simulink model "AttitudeComplementary2"  (Simulink 6.6)
settings: Solver=ode4  StartTime=0.0  StopTime=80  FixedStep=SampleT  RelTol=1e-3
InitFcn:
  | clc
  | Taxi_Var_new
  | failures
  | insInit
  | piccolo_init
values from neighbouring files (symbols this model uses):
  A1 = 0    [Taxi_Var.m]    (also in Taxi_Var_new.m = 0.007)
  Apolar = 0.0899    [Taxi_Var.m]    (also in Taxi_Var_new.m = 0.057)
  APtsamp = 0.005    [failures.m]    (also in piccolo_init.m = 0.05)
  CD0 = 0.0219    [Taxi_Var.m]    (also in Taxi_Var_new.m = 0.022)
  chord = S/span    (= 0.384036716878)    [Taxi_Var.m]    (also in Taxi_Var_new.m = 0.351341681574)
  CL0 = 0.1857    [Taxi_Var.m]    (also in Taxi_Var_new.m = 0.38)
  CLa = 4.6206    [Taxi_Var.m]    (also in Taxi_Var_new.m = 18.5)
  CLa_dot = 1.93    [Taxi_Var.m]    (also in Taxi_Var_new.m = 2.64)
  Clb = -0.0043    [Taxi_Var.m]    (also in Taxi_Var_new.m = -0.06)
  ClDa = 0.1695    [Taxi_Var.m]    (also in Taxi_Var_new.m)
  CLDe = 0.4032    [Taxi_Var.m]    (also in Taxi_Var_new.m = 0.24)
  CLDf = 0.047    [Taxi_Var.m]    (also in Taxi_Var_new.m = 0.4)
  ClDr = 0.0003    [Taxi_Var.m]    (also in Taxi_Var_new.m = 0.055)
  Clp = -0.4425    [Taxi_Var.m]    (also in Taxi_Var_new.m = -0.88)
  CLq = 8.7465    [Taxi_Var.m]    (also in Taxi_Var_new.m = 7.4)
  Clr = 0.0675    [Taxi_Var.m]    (also in Taxi_Var_new.m = 0.04)
  Cm0 = -0.0902    [Taxi_Var.m]    (also in Taxi_Var_new.m = 0.56)
  Cma = -1.3995    [Taxi_Var.m]    (also in Taxi_Var_new.m = -1.58)
  CmDe = -0.9493    [Taxi_Var.m]    (also in Taxi_Var_new.m = -41)
  CmDf = -.021    (= -0.021)    [Taxi_Var.m]    (also in Taxi_Var_new.m)
  Cmq = -10.8760    (= -10.876)    [Taxi_Var.m]    (also in Taxi_Var_new.m = -12)
  Cnb = 0.0281    [Taxi_Var.m]    (also in Taxi_Var_new.m = 0.73)
  CnDa = -0.0031    [Taxi_Var.m]    (also in Taxi_Var_new.m = -0.032)
  CnDr = -0.0882    [Taxi_Var.m]    (also in Taxi_Var_new.m = 0.19)
  Cnp = -0.0695    [Taxi_Var.m]    (also in Taxi_Var_new.m = -0.1)
  Cnr = -0.1045    [Taxi_Var.m]    (also in Taxi_Var_new.m = -0.23)
  CYb = -0.1999    [Taxi_Var.m]    (also in Taxi_Var_new.m = -0.98)
  CYDr = 0.0192    [Taxi_Var.m]    (also in Taxi_Var_new.m = 0.066)
  damax = 25*deg2rad    (= 0.436332312999)    [Taxi_Var.m]    (also in piccolo_init.m)
  damin = -25*deg2rad    (= -0.436332312999)    [Taxi_Var.m]    (also in piccolo_init.m)
  datrim = 0*deg2rad    (= 0)    [Taxi_Var.m]    (also in piccolo_init.m)
  demax = 15*deg2rad    (= 0.261799387799)    [Taxi_Var.m]    (also in piccolo_init.m)
  demin = -15*deg2rad    (= -0.261799387799)    [Taxi_Var.m]    (also in piccolo_init.m)
  detrim = -2.4137*deg2rad    (= -0.0421270121554)    [Taxi_Var.m]    (also in piccolo_init.m = -0.01308996939)
  dfland = 30*deg2rad    (= 0.523598775598)    [Taxi_Var.m]    (also in piccolo_init.m)
  dfmax = 30*deg2rad    (= 0.523598775598)    [Taxi_Var.m]    (also in piccolo_init.m)
  dfmin = 0*deg2rad    (= 0)    [Taxi_Var.m]    (also in piccolo_init.m)
  drmax = 25*deg2rad    (= 0.436332312999)    [Taxi_Var.m]    (also in piccolo_init.m)
  drmin = -25*deg2rad    (= -0.436332312999)    [Taxi_Var.m]    (also in piccolo_init.m)
  drtrim = 0*deg2rad    (= 0)    [Taxi_Var.m]    (also in piccolo_init.m)
  dtmax = 1    [Taxi_Var.m]    (also in piccolo_init.m)
  dtmin = 0    [Taxi_Var.m]    (also in piccolo_init.m)
  dttrim = 0.0725    [Taxi_Var.m]    (also in piccolo_init.m = 0.35)
  Euler_0 = [0; 0; 45]'*pi/180    [Taxi_Var.m]    (also in Taxi_Var_new.m = [0 0 45]'*pi/180)
  heightDown = 0    [insInit.m]
  heightUp = 3000    [insInit.m]
  IdxCmdOrbitRadius = 17    [piccolo_init.m]
  IdxCmdOrbitSense = 18    [piccolo_init.m]
  IdxCmdWp1Alt = 13    [piccolo_init.m]
  IdxCmdWp1Lat = 11    [piccolo_init.m]
  IdxCmdWp1Lon = 12    [piccolo_init.m]
  IdxCmdWp2Alt = 16    [piccolo_init.m]
  IdxCmdWp2Lat = 14    [piccolo_init.m]
  IdxCmdWp2Lon = 15    [piccolo_init.m]
  IdxEstimReserved1 = 4    [piccolo_init.m]
  IdxEstimWEast = 3    [piccolo_init.m]
  IdxEstimWNorth = 2    [piccolo_init.m]
  IdxGainsAltD = 10    [piccolo_init.m]
  IdxGainsAltI = 9    [piccolo_init.m]
  IdxGainsAltP = 8    [piccolo_init.m]
  IdxGainsPdynD = 4    [piccolo_init.m]
  IdxGainsPdynI = 3    [piccolo_init.m]
  IdxGainsPdynP = 2    [piccolo_init.m]
  IdxGainsPitchD = 7    [piccolo_init.m]
  IdxGainsPitchI = 6    [piccolo_init.m]
  IdxGainsPitchP = 5    [piccolo_init.m]
  IdxGainsRollD = 17    [piccolo_init.m]
  IdxGainsRollI = 16    [piccolo_init.m]
  IdxGainsRollP = 15    [piccolo_init.m]
  IdxGainsSlopeElevatorD = 25    [piccolo_init.m]
  IdxGainsSlopeElevatorP = 26    [piccolo_init.m]
  IdxGainsTrackConv = 24    [piccolo_init.m]
  IdxGainsTrackD = 23    [piccolo_init.m]
  IdxGainsTrackI = 22    [piccolo_init.m]
  IdxGainsTrackP = 21    [piccolo_init.m]
  IdxGainsTurnD = 14    [piccolo_init.m]
  IdxGainsTurnI = 13    [piccolo_init.m]
  IdxGainsTurnP = 12    [piccolo_init.m]
  IdxGainsYawD = 20    [piccolo_init.m]
  IdxGainsYawI = 19    [piccolo_init.m]
  IdxGainsYawP = 18    [piccolo_init.m]
  IdxLimitsAileronMax = 11    [piccolo_init.m]
  IdxLimitsAileronMin = 10    [piccolo_init.m]
  IdxLimitsBankMax = 9    [piccolo_init.m]
  IdxLimitsBankMin = 8    [piccolo_init.m]
  IdxLimitsElevatorMax = 13    [piccolo_init.m]
  IdxLimitsElevatorMin = 12    [piccolo_init.m]
  IdxLimitsFlapMax = 19    [piccolo_init.m]
  IdxLimitsFlapMin = 18    [piccolo_init.m]
  IdxLimitsPdynMax = 3    [piccolo_init.m]
  IdxLimitsPdynMin = 2    [piccolo_init.m]
  IdxLimitsRudderMax = 15    [piccolo_init.m]
  IdxLimitsRudderMin = 14    [piccolo_init.m]
  IdxLimitsThrottleMax = 17    [piccolo_init.m]
  IdxLimitsThrottleMin = 16    [piccolo_init.m]
  IdxSensorsAlt = 5    [piccolo_init.m]
  IdxSensorsLat = 3    [piccolo_init.m]
  IdxSensorsLon = 4    [piccolo_init.m]
  IdxSensorsVDown = 8    [piccolo_init.m]
  IdxSensorsVEast = 7    [piccolo_init.m]
  IdxSensorsVNorth = 6    [piccolo_init.m]
  IdxStatesGlobal = 2    [piccolo_init.m]
  IdxStatesManual = 16    [piccolo_init.m]
  IdxStatesMode = 15    [piccolo_init.m]
  ISA_g = 9.815    [Taxi_Var.m]    (also in Taxi_Var_new.m)
  ISA_hmax = 2000    [Taxi_Var.m]    (also in Taxi_Var_new.m)
  ISA_lapse = .0065    (= 0.0065)    [Taxi_Var.m]    (also in Taxi_Var_new.m)
  ISA_P0 = 101325    [Taxi_Var.m]    (also in Taxi_Var_new.m)
  ISA_R = 287    [Taxi_Var.m]    (also in Taxi_Var_new.m)
  ISA_rho0 = 1.225    [Taxi_Var.m]    (also in Taxi_Var_new.m)
  ISA_T0 = 289    [Taxi_Var.m]    (also in Taxi_Var_new.m)
  Ixx = 3.689084    [Taxi_Var.m]    (also in Taxi_Var_new.m = 3.8)
  Iyy = 7.43789    [Taxi_Var.m]    (also in Taxi_Var_new.m = 9.58)
  Izz = 10.22202    [Taxi_Var.m]    (also in Taxi_Var_new.m = 9.68)
  latDown = -100000    [insInit.m]
  latUp = 100000    [insInit.m]
  lonDown = -100000    [insInit.m]
  lonUp = 100000    [insInit.m]
  mass = 22.5    [Taxi_Var.m]    (also in Taxi_Var_new.m = 8.16466266)
  MinThK = 0.075    [Taxi_Var.m]    (also in Taxi_Var_new.m = 0.077)
  ... (+8 more)
undefined symbols (not defined in the file or in its folder): clock, DiscIntNeverNeededParam, Earth, gaind, polesd, WGS84, zerosd
libraries: piccolo_library x60, simulink x51, aerolibconvert2 x14, dspsigops x5, aerolibasang x5, aerolibatmos2 x2, aerolibtransform2 x2, aerolibnav x2, dspmtrx3 x1, aerolibutil x1
(part 1 of 6)
CloseFcn:
  | rtwprivate ssgencode ModelCloseRequest AttitudeComplementary
settings Model: Creator=ASL_Lab  LastModifiedBy=ASL_Lab
settings DebuggingCC: MultiTaskDSMMsg=warning  MultiTaskCondExecSysMsg=none  StrictBusMsg=None
settings HardwareCC: TargetHWDeviceType=32-bit Generic
settings RTWCC: IncludeERTFirstTime=on

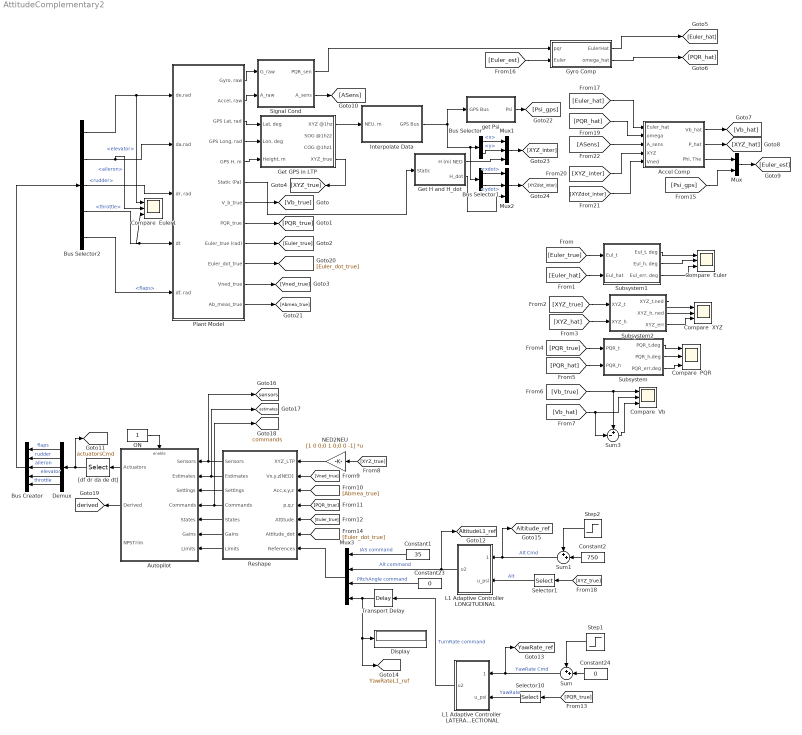
== system AttitudeComplementary2 ==
  Accel Comp : Subsystem
  Autopilot : Subsystem  Orientation=left
  Bus Creator : BusCreator  Orientation=left  Inputs=5
  Bus Selector : BusSelector  OutputSignals=x,y
  Bus Selector1 : BusSelector  OutputSignals=xdot,ydot
  Bus Selector2 : BusSelector  OutputSignals=elevator,aileron,rudder,throttle,flaps
  Compare  Euler : Scope  NumInputPorts=3
      settings: TimeRange=80  YMin=-20~-58.03108808290165~-7.51142166084415  YMax=31.19170984455958~41.45077720207246~7.726417629669186  SaveName=ScopeData20
  Compare  Euler1 : Scope  NumInputPorts=3
      settings: TimeRange=100  YMin=-0.275~-1~0.675  YMax=0.275~1~1  SaveName=ScopeData19
  Compare  PQR : Scope  NumInputPorts=3
      settings: TimeRange=200  YMin=-50~-350000~-450000  YMax=55~450000~350000  SaveName=ScopeData8
  Compare  Vb : Scope  NumInputPorts=3
      settings: TimeRange=1200  YMin=-5~-4.608235729481237~-0.2140564617663046  YMax=35~22.0134426214664~0.2078550324478208  SaveName=ScopeData12
  Compare  XYZ : Scope  NumInputPorts=3
      settings: TimeRange=70  YMin=-1000~-1000~-2.5  YMax=1200~1200~4  SaveName=ScopeData2
  Constant1 : Constant  Orientation=left  Value=35
  Constant2 : Constant  Orientation=left  Value=750
  Constant23 : Constant  Orientation=left  Value=0
  Constant24 : Constant  Orientation=left  Value=0
  Demux : Demux  Orientation=left  Outputs=5
  Display : Display
  Get GPS in LTP : Subsystem
  "Get H and H_dot " : Subsystem
  Gyro Comp : Subsystem
  Interpolate Data : Subsystem
  L1 Adaptive Controller LATERAL-DIRECTIONAL : Subsystem  Orientation=left  mask{gamma=-2000, m=4, omega=2, Pbound=.1, L1ONOFF=0}
      mask prompts: gamma "L1 gain"; m "state predictor (m)"; omega "low-pass filter (omega)"; Pbound "projection bounds"; L1ONOFF "L1 switch"
  L1 Adaptive Controller LONGITUDINAL : Subsystem  Orientation=left  mask{gamma=-1, m=4, omega=1, Pbound=50, L1ONOFF=0}
      mask prompts: gamma "L1 gain"; m "state predictor (m)"; omega "low-pass filter (omega)"; Pbound "projection bounds"; L1ONOFF "L1 switch"
  Mux : Mux  Inputs=2
  Mux1 : Mux  Inputs=3
  Mux2 : Mux  Inputs=3
  Mux3 : Mux  Orientation=left
  NED2NEU : Gain  Orientation=left  Gain=[1 0 0;0 1 0;0 0 -1]  Multiplication=Matrix(K*u)  SaturateOnIntegerOverflow=on
  ON : Constant
  Plant Model : Subsystem
  Reshape : Subsystem  Orientation=left
  Selector1 : Selector  Orientation=left  IndexOptions=Index vector (dialog)  Indices=3  OutputSizes=1  InputPortWidth=3
  Selector10 : Selector  Orientation=left  IndexOptions=Index vector (dialog)  Indices=3  OutputSizes=1  InputPortWidth=3
  Signal Cond : Subsystem
  Step1 : Step  Orientation=left  Time=2  After=0  SampleTime=0
  Step2 : Step  Orientation=left  Time=35  After=-250  SampleTime=0
  Subsystem : Subsystem
  Subsystem1 : Subsystem
  Subsystem2 : Subsystem
  Sum : Sum  Orientation=left  Inputs=++|  SaturateOnIntegerOverflow=on
  Sum1 : Sum  Orientation=left  Inputs=++|  SaturateOnIntegerOverflow=on
  Sum3 : Sum  Inputs=+-|
  Transport Delay : TransportDelay  Orientation=left  DelayTime=tdelay
  "[df dr da de dt]" : Selector  Orientation=left  IndexOptions=Index vector (dialog)  Indices=[10 6 2 4 8]  OutputSizes=[(-2)]  InputPortWidth=12
  get Psi : Subsystem
  tag scope: AltitudeL1_ref=global, Altitude_ref=global, YawRateL1_ref=global, YawRate_ref=global, actuatorsCmd=global, commands=global, derived=global, estimates=global, sensors=global
  wires:
  Plant Model/1("Gyro, raw") -> Signal Cond/1(G_raw)
  Plant Model/2("Accel, raw") -> Signal Cond/2(A_raw)
  Plant Model/3("GPS Lat, rad") -> Get GPS in LTP/1("Lat, deg")
  Plant Model/5("GPS H, m") -> Get GPS in LTP/3("Height, m")
  Plant Model/4("GPS Long, rad") -> Get GPS in LTP/2("Lon, deg")
  Signal Cond/1(PQR_sen) -> Gyro Comp/1(pqr)
  Gyro Comp/1(EulerHat) -> [Euler_hat]
  Accel Comp/3("Phi, The") -> Mux/1
  Get GPS in LTP/1(XYZ @1hz) -> Interpolate Data/1(NEU. m)
  Gyro Comp/2(omega_hat) -> [PQR_hat]
  Bus Selector/1 -> Mux1/1  "<x>"
  Bus Selector/2 -> Mux1/2  "<y>"
  Bus Selector1/1 -> Mux2/1  "<xdot>"
  Bus Selector1/2 -> Mux2/2  "<ydot>"
  Plant Model/7(V_b_true) -> [Vb_true]
  Plant Model/8(PQR_true) -> [PQR_true]
  Plant Model/9(Euler_true (rad)) -> [Euler_true]
  Plant Model/11(Vned_true) -> [Vned_true]
  Accel Comp/1(Vb_hat) -> [Vb_hat]
  Accel Comp/2(P_hat) -> [XYZ_hat]
  Subsystem1/1("Eul_t, deg") -> Compare  Euler/1
  Subsystem1/2("Eul_h, deg") -> Compare  Euler/2
  Subsystem1/3("Eul_err, deg") -> Compare  Euler/3
  [XYZ_true] -> Subsystem2/1(XYZ_t)
  [XYZ_hat] -> Subsystem2/2(XYZ_h)
  Subsystem/1(PQR_t,deg) -> Compare  PQR/1
  Subsystem/2(PQR_h,deg) -> Compare  PQR/2
  Subsystem/3(PQR_err,deg) -> Compare  PQR/3
  [Vb_true] -> Compare  Vb/1, Sum3/1
  [Vb_hat] -> Sum3/2, Compare  Vb/2
  Sum3/1 -> Compare  Vb/3
  Get GPS in LTP/4(XYZ_true) -> [XYZ_true]
  [PQR_true] -> Subsystem/1(PQR_t)
  [PQR_hat] -> Subsystem/2(PQR_h)
  [Euler_true] -> Subsystem1/1(Eul_t)
  [Euler_hat] -> Subsystem1/2(Eul_hat)
  Subsystem2/1(XYZ_t,ned) -> Compare  XYZ/1
  Subsystem2/2("XYZ_h, ned") -> Compare  XYZ/2
  Subsystem2/3(XYZ_err) -> Compare  XYZ/3
  "Get H and H_dot "/1(H (m) NED) -> Mux1/3
  "Get H and H_dot "/2(H_dot) -> Mux2/3
  [XYZ_true] -> NED2NEU/1
  [Vned_true] -> Reshape/2(Vx,y,z[NED])
  [Abmea_true] -> Reshape/3(Acc,x,y,z)
  [PQR_true] -> Reshape/4(p,q,r)
  Reshape/1(Sensors) -> Autopilot/1(Sensors), [sensors]
  Reshape/2(Estimates) -> Autopilot/2(Estimates), [estimates]
  Reshape/3(Settings) -> Autopilot/3(Settings)
  Reshape/4(Commands) -> Autopilot/4(Commands), [commands]
  Reshape/5(States) -> Autopilot/5(States)
  Reshape/6(Gains) -> Autopilot/6(Gains)
  Reshape/7(Limits) -> Autopilot/7(Limits)
  ON/1 -> Autopilot/Enable
  Autopilot/1(Actuators) -> "[df dr da de dt]"/1
  "[df dr da de dt]"/1 -> Demux/1, [actuatorsCmd]
  [Euler_true] -> Reshape/5(Attitude)
  [Euler_dot_true] -> Reshape/6(Attitude_dot)
  Autopilot/2(Derived) -> [derived]
  Constant1/1 -> Mux3/1  "IAS command"
  L1 Adaptive Controller LONGITUDINAL/1(u2) -> [AltitudeL1_ref], Mux3/2  "Alt command"
  Constant23/1 -> Mux3/3  "PitchAngle command"
  L1 Adaptive Controller LATERAL-DIRECTIONAL/1(u2) -> Transport Delay/1  "TurnRate command"
  Mux3/1 -> Reshape/7(References)
  Sum/1 -> L1 Adaptive Controller LATERAL-DIRECTIONAL/1(u_psi_c), [YawRate_ref]  "YawRate Cmd"
  [PQR_true] -> Selector10/1
  Selector10/1 -> L1 Adaptive Controller LATERAL-DIRECTIONAL/2(u_psi)  "YawRate"
  Constant24/1 -> Sum/2
  Step1/1 -> Sum/1
  Transport Delay/1 -> Mux3/4, Display/1, [YawRateL1_ref]
  Sum1/1 -> [Altitude_ref], L1 Adaptive Controller LONGITUDINAL/1(u_psi_c)  "Alt Cmd"
  Constant2/1 -> Sum1/2
  Step2/1 -> Sum1/1
  [XYZ_true] -> Selector1/1
  Selector1/1 -> L1 Adaptive Controller LONGITUDINAL/2(u_psi)  "Alt"
  Demux/1 -> Bus Creator/1  "flaps"
  Demux/2 -> Bus Creator/2  "rudder"
  Demux/3 -> Bus Creator/3  "aileron"
  Demux/4 -> Bus Creator/4  "elevator"
  Demux/5 -> Bus Creator/5  "throttle"
  Bus Creator/1 -> Bus Selector2/1
  Bus Selector2/1 -> Plant Model/1(de,rad), Compare  Euler1/1  "<elevator>"
  Bus Selector2/2 -> Plant Model/2(da,rad), Compare  Euler1/2  "<aileron>"
  Bus Selector2/3 -> Plant Model/3("dr, rad")  "<rudder>"
  Bus Selector2/4 -> Compare  Euler1/3, Plant Model/4(dt)  "<throttle>"
  Bus Selector2/5 -> Plant Model/5("df, rad")  "<flaps>"
  Plant Model/10(Euler_dot_true) -> [Euler_dot_true]
  Plant Model/12(Ab_meas_true) -> [Abmea_true]
  Mux/1 -> [Euler_est]
  Plant Model/6(Static (Pa)) -> "Get H and H_dot "/1(Static)
  Interpolate Data/1(GPS Bus) -> Bus Selector/1, Bus Selector1/1, get Psi/1(GPS Bus)
  get Psi/1(Psi) -> [Psi_gps]
  Mux1/1 -> [XYZ_inter]
  Mux2/1 -> [XYZdot_inter]
  [Psi_gps] -> Mux/2
  [Euler_est] -> Gyro Comp/2(Euler)
  [Euler_hat] -> Accel Comp/1(Euler_hat)
  [PQR_hat] -> Accel Comp/2(omega)
  [XYZ_inter] -> Accel Comp/4(XYZ)
  [XYZdot_inter] -> Accel Comp/5(Vned)
  Signal Cond/2(A_sens) -> [ASens]
  [ASens] -> Accel Comp/3(A_sens)
  NED2NEU/1 -> Reshape/1(XYZ_LTP)

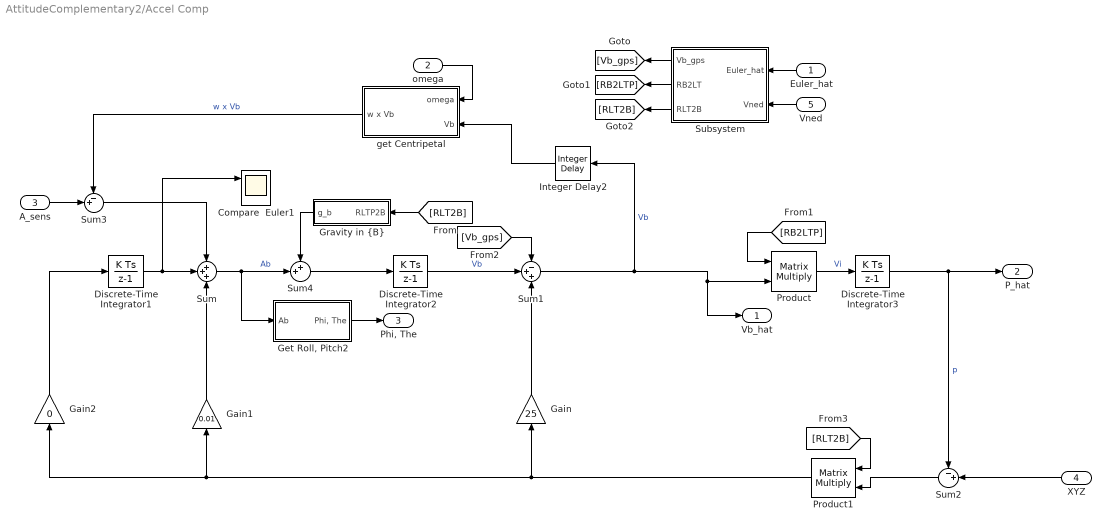
== system AttitudeComplementary2/Accel Comp ==
  Euler_hat : Inport  Orientation=left
  omega : Inport  Port=2
  A_sens : Inport  Port=3
  XYZ : Inport  Orientation=left  Port=4
  Vned : Inport  Orientation=left  Port=5
  Compare  Euler1 : Scope  NumInputPorts=3
      settings: TimeRange=80  YMin=-20~-200~-7.51142166084415  YMax=60~200~7.726417629669186  SaveName=ScopeData23
  Discrete-Time Integrator1 : DiscreteIntegrator  SampleTime=SampleT  ICPrevOutput=DiscIntNeverNeededParam  ICPrevScaledInput=DiscIntNeverNeededParam
  Discrete-Time Integrator2 : DiscreteIntegrator  InitialCondition=Vb_0  SampleTime=SampleT  ICPrevOutput=DiscIntNeverNeededParam  ICPrevScaledInput=DiscIntNeverNeededParam
  Discrete-Time Integrator3 : DiscreteIntegrator  InitialCondition=[Pos_0(1) Pos_0(2) -Pos_0(3)]  SampleTime=SampleT  ICPrevOutput=DiscIntNeverNeededParam  ICPrevScaledInput=DiscIntNeverNeededParam
  Gain : Gain  Orientation=up  Gain=25
  Gain1 : Gain  Orientation=up  Gain=0.01
  Gain2 : Gain  Orientation=up  Gain=0
  "Get Roll, Pitch2" : Subsystem
  "Gravity in {B}" : Subsystem  Orientation=left
  Integer Delay2 : simulink/Discrete/Integer Delay  Orientation=left  vinit=0.0  samptime=-1  NumDelays=1
  Product : Product  Multiplication=Matrix(*)  RndMeth=Zero
  Product1 : Product  Orientation=left  Multiplication=Matrix(*)  RndMeth=Zero
  Subsystem : Subsystem  Orientation=left
  Sum : Sum  Inputs=+++
  Sum1 : Sum  Inputs=-++
  Sum2 : Sum  Orientation=left  Inputs=-+|
  Sum3 : Sum  Inputs=-+|
  Sum4 : Sum  Inputs=++|
  get Centripetal : Subsystem  Orientation=left
  Vb_hat : Outport
  P_hat : Outport  Port=2
  "Phi, The" : Outport  Port=3
  wires:
  Sum2/1 -> Product1/2
  Discrete-Time Integrator3/1 -> Sum2/1, P_hat/1  "p"
  Discrete-Time Integrator1/1 -> Sum/2, Compare  Euler1/1
  Discrete-Time Integrator2/1 -> Sum1/2  "Vb"
  "Get Roll, Pitch2"/1("Phi, The") -> "Phi, The"/1
  A_sens/1 -> Sum3/2
  omega/1 -> get Centripetal/1(omega)
  Euler_hat/1 -> Subsystem/1(Euler_hat)
  Vned/1 -> Subsystem/2(Vned)
  Product/1 -> Discrete-Time Integrator3/1  "Vi"
  Sum1/1 -> Integer Delay2/1, Product/2, Vb_hat/1  "Vb"
  XYZ/1 -> Sum2/2
  Subsystem/1(Vb_gps) -> [Vb_gps]
  Subsystem/2(RB2LT) -> [RB2LTP]
  Subsystem/3(RLT2B) -> [RLT2B]
  [RLT2B] -> "Gravity in {B}"/1(RLTP2B)
  [RB2LTP] -> Product/1
  [Vb_gps] -> Sum1/1
  [RLT2B] -> Product1/1
  Product1/1 -> Gain2/1, Gain1/1, Gain/1
  Gain2/1 -> Discrete-Time Integrator1/1
  Gain1/1 -> Sum/3
  Gain/1 -> Sum1/3
  Sum3/1 -> Sum/1
  Sum4/1 -> Discrete-Time Integrator2/1
  "Gravity in {B}"/1(g_b) -> Sum4/1
  Sum/1 -> Sum4/2, "Get Roll, Pitch2"/1(Ab)  "Ab"
  Integer Delay2/1 -> get Centripetal/2(Vb)
  get Centripetal/1(w x Vb) -> Sum3/1  "w x Vb"

== system AttitudeComplementary2/Autopilot ==
  Sensors : Inport  PortDimensions=SizeSensors
  Estimates : Inport  Port=2  PortDimensions=SizeEstim
  Settings : Inport  Port=3  PortDimensions=SizeSet
  Commands : Inport  Port=4  PortDimensions=SizeCmd
  States : Inport  Port=5  PortDimensions=SizeStates
  Gains : Inport  Port=6  PortDimensions=SizeGains
  Limits : Inport  Port=7  PortDimensions=SizeLimits
  Autopilot Enable : EnablePort  StatesWhenEnabling=reset
  Air System Vector Inputs : piccolo_library/Flight Mechanics/Air System Vector Inputs  SystemSampleTime=-1  tsamp=APtsamp
  Altitude Control Vector Inputs : Subsystem  AncestorBlock=piccolo_library/Controllers/Longitudinal/Altitude Control Vector Inputs  mask(Altitude controller){tsamp=APtsamp}
      mask prompts: tsamp "Sample time:"
      mask help: The system computes the throttle command required for maintaining a specified altitude.
  Demux{,1..6} (7 alike) : Demux  Outputs=7
  Flap Control Vector Inputs : Subsystem  mask(Flap controller){tsamp=APtsamp}
      mask prompts: tsamp "Sample time:"
      mask help: The system provides the flap command.
  Gain : Gain  SaturateOnIntegerOverflow=on
  Gain1 : Gain  SaturateOnIntegerOverflow=on
  Guidance & Navigation Vector Input : Subsystem  AncestorBlock=piccolo_library/Controllers/Guidance/Guidance & Navigation Vector Input  mask(Guidance and Navigation){tsamp=1, aptsamp=APtsamp}
      mask prompts: tsamp "Guidance sample time:"; aptsamp "Autopilot sample time:"
      mask help: Steer the airplane to track a flightplan or to loiter around a single waypoint.
  Mux : Mux  Inputs=12
  Mux1 : Mux  Inputs=5
  Mux2 : Mux  Inputs=7
  Pitch Control  Vector Inputs : Subsystem  AncestorBlock="piccolo_library/Controllers/Longitudinal/Pitch Control  Vector Inputs"  mask(Pitch Control){tsamp=APtsamp}
      mask prompts: tsamp "Sample time:"
      mask help: The pitch controller includes pitch angle hold, dynamic pressure hold, and turn compensation.
  Reserved Outputs : Constant  Value=0
  Roll Control Vector Inputs : Subsystem  AncestorBlock=piccolo_library/Controllers/Lateral/Roll Control Vector Inputs  mask(Roll Control){tsamp=APtsamp}
      mask prompts: tsamp "Sample time:"
      mask help: Roll controller using bank angle hold and turn rate hold.
  Yaw Control Vector Inputs : Subsystem  AncestorBlock=piccolo_library/Controllers/Lateral/Yaw Control Vector Inputs  mask(Yaw Control){tsamp=APtsamp}
      mask prompts: tsamp "Sample time:"
      mask help: Yaw controller using PID loops and actuator output saturation.
  Actuators : Outport  OutDataType=fixdt(1,16,0)  OutScaling=[]
  Derived : Outport  Port=2  OutDataType=fixdt(1,16,0)  OutScaling=[]
  NPSTrim : Outport  Port=3  OutDataType=fixdt(1,16,0)  OutScaling=[]
  wires:
  Mux/1 -> Gain/1, NPSTrim/1
  Mux1/1 -> Roll Control Vector Inputs/8(Derived), Altitude Control Vector Inputs/8(Derived), Pitch Control  Vector Inputs/8(Derived), Guidance & Navigation Vector Input/8(Derived), Yaw Control Vector Inputs/8(Derived), Air System Vector Inputs/8, Flap Control Vector Inputs/8(Derived), Gain1/1
  Roll Control Vector Inputs/1(Actuator) -> Mux/2
  Pitch Control  Vector Inputs/1(Actuator) -> Mux/4
  Altitude Control Vector Inputs/1(Actuator) -> Mux/8
  Sensors/1 -> Mux2/1
  Estimates/1 -> Mux2/2
  Settings/1 -> Mux2/3
  Commands/1 -> Mux2/4
  States/1 -> Mux2/5
  Gains/1 -> Mux2/6
  Limits/1 -> Mux2/7
  Demux/1 -> Altitude Control Vector Inputs/1(Sensors)
  Demux/2 -> Altitude Control Vector Inputs/2(Estimates)
  Demux/3 -> Altitude Control Vector Inputs/3(Settings)
  Demux/4 -> Altitude Control Vector Inputs/4(Commands)
  Demux/5 -> Altitude Control Vector Inputs/5(States)
  Demux/6 -> Altitude Control Vector Inputs/6(Gains)
  Demux/7 -> Altitude Control Vector Inputs/7(Limits)
  Demux1/1 -> Roll Control Vector Inputs/1(Sensors)
  Demux1/2 -> Roll Control Vector Inputs/2(Estimates)
  Demux1/3 -> Roll Control Vector Inputs/3(Settings)
  Demux1/4 -> Roll Control Vector Inputs/4(Commands)
  Demux1/5 -> Roll Control Vector Inputs/5(States)
  Demux1/6 -> Roll Control Vector Inputs/6(Gains)
  Demux1/7 -> Roll Control Vector Inputs/7(Limits)
  Demux2/1 -> Pitch Control  Vector Inputs/1(Sensors)
  Demux2/2 -> Pitch Control  Vector Inputs/2(Estimates)
  Demux2/3 -> Pitch Control  Vector Inputs/3(Settings)
  Demux2/4 -> Pitch Control  Vector Inputs/4(Commands)
  Demux2/5 -> Pitch Control  Vector Inputs/5(States)
  Demux2/6 -> Pitch Control  Vector Inputs/6(Gains)
  Demux2/7 -> Pitch Control  Vector Inputs/7(Limits)
  Demux3/1 -> Guidance & Navigation Vector Input/1(Sensors)
  Demux3/2 -> Guidance & Navigation Vector Input/2(Estimates)
  Demux3/3 -> Guidance & Navigation Vector Input/3(Settings)
  Demux3/4 -> Guidance & Navigation Vector Input/4(Commands)
  Demux3/5 -> Guidance & Navigation Vector Input/5(States)
  Demux3/6 -> Guidance & Navigation Vector Input/6(Gains)
  Demux3/7 -> Guidance & Navigation Vector Input/7(Limits)
  Demux4/1 -> Yaw Control Vector Inputs/1(Sensors)
  Demux4/2 -> Yaw Control Vector Inputs/2(Estimates)
  Demux4/3 -> Yaw Control Vector Inputs/3(Settings)
  Demux4/4 -> Yaw Control Vector Inputs/4(Commands)
  Demux4/5 -> Yaw Control Vector Inputs/5(States)
  Demux4/6 -> Yaw Control Vector Inputs/6(Gains)
  Demux4/7 -> Yaw Control Vector Inputs/7(Limits)
  Demux5/1 -> Air System Vector Inputs/1
  Demux5/2 -> Air System Vector Inputs/2
  Demux5/3 -> Air System Vector Inputs/3
  Demux5/4 -> Air System Vector Inputs/4
  Demux5/5 -> Air System Vector Inputs/5
  Demux5/6 -> Air System Vector Inputs/6
  Demux5/7 -> Air System Vector Inputs/7
  Mux2/1 -> Demux1/1, Demux/1, Demux2/1, Demux3/1, Demux4/1, Demux5/1, Demux6/1
  Reserved Outputs/1 -> Mux/11, Mux/9, Mux/7, Mux/1, Mux/3, Mux/5, Mux/12
  Yaw Control Vector Inputs/1(Actuator) -> Mux/6
  Flap Control Vector Inputs/1(Actuator) -> Mux/10
  Demux6/1 -> Flap Control Vector Inputs/1(Sensors)
  Demux6/2 -> Flap Control Vector Inputs/2(Estimates)
  Demux6/3 -> Flap Control Vector Inputs/3(Settings)
  Demux6/4 -> Flap Control Vector Inputs/4(Commands)
  Demux6/5 -> Flap Control Vector Inputs/5(States)
  Demux6/6 -> Flap Control Vector Inputs/6(Gains)
  Demux6/7 -> Flap Control Vector Inputs/7(Limits)
  Air System Vector Inputs/1 -> Mux1/1
  Roll Control Vector Inputs/2(Param) -> Mux1/2
  Pitch Control  Vector Inputs/2(Param) -> Mux1/3
  Guidance & Navigation Vector Input/1(Param) -> Mux1/4
  Altitude Control Vector Inputs/2(Param) -> Mux1/5
  Gain/1 -> Actuators/1
  Gain1/1 -> Derived/1

== system AttitudeComplementary2/Get GPS in LTP ==
  "Lat, deg" : Inport
  "Lon, deg" : Inport  Port=2
  "Height, m" : Inport  Port=3
  Angle Conversion : aerolibconvert2/Angle Conversion  SystemSampleTime=-1  IU=rad  OU=deg
  Angle Conversion1 : aerolibconvert2/Angle Conversion  SystemSampleTime=-1  IU=rad  OU=deg
  Angle Conversion2 : aerolibconvert2/Angle Conversion  SystemSampleTime=-1  IU=rad  OU=deg
  Constant : Constant  Orientation=left  Value=[0 , 37.0004768371582, -122.061897277832]
  Demux : Demux  Outputs=3
  Demux1 : Demux  Outputs=3
  Discrete Derivative : simulink/Discrete/Discrete Derivative  SystemSampleTime=-1  gainval=1.0  ICPrevScaledInput=0.0  OutDataType=sfix(16)  OutScaling=2^-10  DoSatur=off
  Fcn : Fcn  Expr=sqrt(u(1)^2+u(2)^2+u(3)^2)
  Geod2LTP2 : Subsystem
      mask Description:
      | This block provides transformation of the Geodetic coordinates
      | to the LTP coorinate system. The block uses two consecutive transformations
      | (Geodetic -> ECEF ->LTP).
      | Geodetic coordinates of the LTP origin should also be predetermined.
      mask Help: Oops!
      mask Display: plot(0,0,100,100,[45,40,35,40,40],[85,95,85,95,40],[85,95,85,95,40],[35,40,45,40,40],[60,40,10,20,10,14],[70,40,10,13,10,20],[56,45],[70,70],[60,60],[50,60],[60,60],[30,40],[50,60],[20,20],[30,40],[20,20],[45,55],[35,25],[75,65],[35,25])
  Mux : Mux  Inputs=3
  NED2NEU : Gain  Gain=[1 0 0;0 1 0;0 0 -1]  Multiplication=Matrix(K*u)  SaturateOnIntegerOverflow=on
  Reshape1 : Reshape
  Sim Latency : Subsystem
  Sim Latency3 : Subsystem
  Sim Latency4 : Subsystem
  Sim Latency5 : Subsystem
  Sim Latency6 : Subsystem
  Trigonometric Function : Trigonometry  Operator=atan2
  XYZ @1hz : Outport
  SOG @1hz2 : Outport  Port=2
  COG @1hz1 : Outport  Port=3
  XYZ_true : Outport  Port=4
  wires:
  Constant/1 -> Geod2LTP2/1("Height, Lat, Lon Initials from GPS")
  Geod2LTP2/1("NEU, m") -> Demux1/1, Discrete Derivative/1, Reshape1/1
  "Lat, deg"/1 -> Angle Conversion1/1
  "Lon, deg"/1 -> Angle Conversion2/1
  "Height, m"/1 -> Geod2LTP2/4(Hight,m(GPS))
  Fcn/1 -> Sim Latency6/1(Fast Data)
  Demux/2 -> Trigonometric Function/1
  Demux/1 -> Trigonometric Function/2
  Trigonometric Function/1 -> Angle Conversion/1
  Angle Conversion/1 -> Sim Latency5/1(Fast Data)
  Discrete Derivative/1 -> Demux/1, Fcn/1
  Mux/1 -> XYZ @1hz/1
  Angle Conversion1/1 -> Geod2LTP2/2("Lat, deg(GPS)")
  Angle Conversion2/1 -> Geod2LTP2/3("Lon, deg(GPS)")
  Demux1/1 -> Sim Latency/1(Fast Data)
  Demux1/2 -> Sim Latency3/1(Fast Data)
  Demux1/3 -> Sim Latency4/1(Fast Data)
  Sim Latency/1(1Hz Data) -> Mux/1
  Sim Latency3/1(1Hz Data) -> Mux/2
  Sim Latency4/1(1Hz Data) -> Mux/3
  Sim Latency5/1(1Hz Data) -> COG @1hz1/1
  Sim Latency6/1(1Hz Data) -> SOG @1hz2/1
  Reshape1/1 -> NED2NEU/1
  NED2NEU/1 -> XYZ_true/1

== system AttitudeComplementary2/Get H and H_dot  ==
  Static : Inport
  Discrete Derivative : simulink/Discrete/Discrete Derivative  SystemSampleTime=-1  gainval=1.0  ICPrevScaledInput=-0.6  OutDataType=sfix(16)  OutScaling=2^-10  DoSatur=off
  Gain : Gain  Gain=-1
  Pressure Altitude : aerolibatmos2/Pressure Altitude  SystemSampleTime=-1  units=Metric (MKS)  action=Warning
  H (m) NED : Outport
  H_dot : Outport  Port=2
  wires:
  Pressure Altitude/1 -> Gain/1
  Gain/1 -> Discrete Derivative/1, H (m) NED/1
  Discrete Derivative/1 -> H_dot/1
  Static/1 -> Pressure Altitude/1

== system AttitudeComplementary2/Gyro Comp ==
  pqr : Inport
  Euler : Inport  Orientation=left  Port=2
  3vector LPF : Subsystem  mask{flpf=5}
      mask prompts: flpf "LowPass Freq"
      mask Display: droots([],-flpf,flpf)
  Constant : Constant  Value=[1 0 0]
  Discrete-Time Integrator1 : DiscreteIntegrator  SampleTime=SampleT  ICPrevOutput=DiscIntNeverNeededParam  ICPrevScaledInput=DiscIntNeverNeededParam
  Discrete-Time Integrator2 : DiscreteIntegrator  InitialCondition=PQR_0  SampleTime=SampleT  ICPrevOutput=DiscIntNeverNeededParam  ICPrevScaledInput=DiscIntNeverNeededParam
  Discrete-Time Integrator3 : DiscreteIntegrator  InitialCondition=Euler_0  SampleTime=SampleT  ICPrevOutput=DiscIntNeverNeededParam  ICPrevScaledInput=DiscIntNeverNeededParam
  Embedded MATLAB Function : Stateflow chart
  Gain : Gain  Orientation=up  Gain=3
  Gain1 : Gain  Orientation=up  Gain=0.5
  Gain2 : Gain  Orientation=up  Gain=0.01
  Integer Delay : simulink/Discrete/Integer Delay  Orientation=left  vinit=0.0  samptime=-1  NumDelays=1
  Scope1 : Scope
      settings: YMin=-0.08  YMax=0.035  SaveName=ScopeData28
  Slider Gain : simulink/Math Operations/Slider Gain  SystemSampleTime=-1  low=0  gain=0  high=0.09
  Sum : Sum  Inputs=+++
  Sum1 : Sum  Inputs=|++
  Sum2 : Sum  Orientation=left  Inputs=-+|
  Sum3 : Sum  Inputs=|++
  EulerHat : Outport
  omega_hat : Outport  Port=2
  wires:
  Discrete-Time Integrator2/1 -> Sum/2
  Sum1/1 -> Discrete-Time Integrator2/1
  Discrete-Time Integrator1/1 -> Sum1/1, Scope1/1
  Gain/1 -> Sum/3
  Gain1/1 -> Sum1/2
  Gain2/1 -> Discrete-Time Integrator1/1
  Discrete-Time Integrator3/1 -> EulerHat/1, Sum2/1, Integer Delay/1
  Euler/1 -> Sum2/2
  Sum2/1 -> Gain2/1, Gain1/1, Gain/1
  Sum/1 -> Embedded MATLAB Function/2(pqr), 3vector LPF/1(In1)
  Embedded MATLAB Function/1(lamDot) -> Discrete-Time Integrator3/1
  Integer Delay/1 -> Embedded MATLAB Function/1(lam)
  pqr/1 -> Sum3/1
  Sum3/1 -> Sum/1
  Constant/1 -> Slider Gain/1
  Slider Gain/1 -> Sum3/2
  3vector LPF/1(Out1) -> omega_hat/1

== system AttitudeComplementary2/Interpolate Data ==
  NEU. m : Inport
  Bus Creator : BusCreator  Inputs=9
  Demux : Demux  Outputs=3
  Saturation : Saturate  UpperLimit=latUp  LowerLimit=latDown
  Saturation1 : Saturate  UpperLimit=lonUp  LowerLimit=lonDown
  Saturation2 : Saturate  UpperLimit=heightUp  LowerLimit=heightDown
  Subsystem : Subsystem
  Subsystem1 : Subsystem
  Subsystem2 : Subsystem
  GPS Bus : Outport
  wires:
  Demux/1 -> Saturation/1
  Demux/2 -> Saturation1/1
  Demux/3 -> Saturation2/1
  Saturation/1 -> Subsystem/1(data)
  Saturation1/1 -> Subsystem1/1(data)
  Saturation2/1 -> Subsystem2/1(data)
  Subsystem/1(Est) -> Bus Creator/1  "x"
  Subsystem/2(dotEst) -> Bus Creator/2  "xdot"
  Subsystem/3(ddotEst) -> Bus Creator/3  "xddot"
  Subsystem1/1(Est) -> Bus Creator/4  "y"
  Subsystem1/2(dotEst) -> Bus Creator/5  "ydot"
  Subsystem1/3(ddotEst) -> Bus Creator/6  "yddot"
  Subsystem2/1(Est) -> Bus Creator/7  "z"
  Subsystem2/2(dotEst) -> Bus Creator/8  "zdot"
  Subsystem2/3(ddotEst) -> Bus Creator/9  "zddot"
  Bus Creator/1 -> GPS Bus/1
  NEU. m/1 -> Demux/1

== system AttitudeComplementary2/L1 Adaptive Controller LATERAL-DIRECTIONAL ==
  u_psi_c : Inport
  u_psi : Inport  Port=2
  Display : Display
  Mux2 : Mux  Inputs=2
  PF Yaw Channel L1 Augmentation : Subsystem  Orientation=left
  Scope1 : Scope  NumInputPorts=2
      settings: YMin=0.0999875~-4.5e-005  YMax=0.100045~1.25e-005  SaveName=ScopeData28
  Sum1 : Sum  Inputs=-+|
  Sum2 : Sum  Inputs=-+|
  u2 : Outport
  wires:
  u_psi/1 -> PF Yaw Channel L1 Augmentation/1(u_psi), Mux2/2, Sum2/1
  PF Yaw Channel L1 Augmentation/1(C_sighat_2) -> Sum1/1, Display/1  "L1 augmentation"
  u_psi_c/1 -> Sum1/2, Mux2/1, Sum2/2
  Sum1/1 -> u2/1, PF Yaw Channel L1 Augmentation/2(u2)
  Mux2/1 -> Scope1/1
  Sum2/1 -> Scope1/2

== system AttitudeComplementary2/L1 Adaptive Controller LONGITUDINAL ==
  u_psi_c : Inport
  u_psi : Inport  Port=2
  Display : Display
  Mux2 : Mux  Inputs=2
  PF Yaw Channel L1 Augmentation : Subsystem  Orientation=left
  Scope1 : Scope  NumInputPorts=2
      settings: YMin=0.0999875~-4.5e-005  YMax=0.100045~1.25e-005  SaveName=ScopeData28
  Sum1 : Sum  Inputs=-+|
  Sum2 : Sum  Inputs=-+|
  u2 : Outport
  wires:
  Sum2/1 -> Scope1/2
  Mux2/1 -> Scope1/1
  Sum1/1 -> PF Yaw Channel L1 Augmentation/2(u2), u2/1
  u_psi_c/1 -> Sum2/2, Mux2/1, Sum1/2
  PF Yaw Channel L1 Augmentation/1(C_sighat_2) -> Display/1, Sum1/1  "L1 augmentation"
  u_psi/1 -> Sum2/1, Mux2/2, PF Yaw Channel L1 Augmentation/1(u_psi)

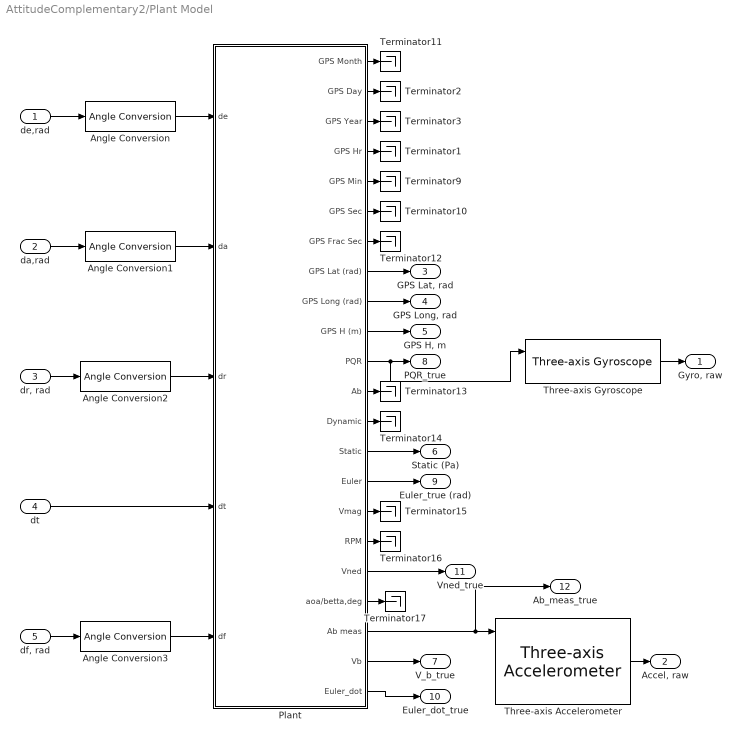
== system AttitudeComplementary2/Plant Model ==
  de,rad : Inport
  da,rad : Inport  Port=2
  "dr, rad" : Inport  Port=3
  dt : Inport  Port=4
  "df, rad" : Inport  Port=5
  Angle Conversion{,1..3} (4 alike) : aerolibconvert2/Angle Conversion  SystemSampleTime=-1  IU=rad  OU=deg
  Plant : Subsystem
  Terminator{1..3,9..17} (12 alike) : Terminator
  Three-axis Accelerometer : aerolibnav/Three-axis Accelerometer  SystemSampleTime=-1  units=Metric (MKS)  acc=[0 0 0]  gtype=off  dtype_a=on  w_a=190  z_a=0.707  a_sf_cc=[-41 0 0; 0 41 0; 0 0 -43]  a_bias=[2015 2018 2006]  a_rand=on  a_seeds=[23093 23094 23095]  a_pow=[0.008 0.008 0.008]  a_sat="[-inf  -inf  -inf  inf inf inf]"  a_Ts=SampleT
  Three-axis Gyroscope : aerolibnav/Three-axis Gyroscope  SystemSampleTime=-1  dtype_g=on  w_g=190  z_g=0.707  g_sf_cc=[-142 0 0; 0 142 0; 0 0 235]  g_bias=[1866 1981 2042]  g_sen=[0 0 0]  g_rand=on  g_seeds=[23093 23094 23095]  g_pow=[0.008 0.008 0.008]  g_sat="[-inf  -inf  -inf  inf inf inf]"  g_Ts=SampleT
  "Gyro, raw" : Outport
  "Accel, raw" : Outport  Port=2
  "GPS Lat, rad" : Outport  Port=3
  "GPS Long, rad" : Outport  Port=4
  "GPS H, m" : Outport  Port=5
  Static (Pa) : Outport  Port=6
  V_b_true : Outport  Port=7
  PQR_true : Outport  Port=8
  Euler_true (rad) : Outport  Port=9
  Euler_dot_true : Outport  Port=10
  Vned_true : Outport  Port=11
  Ab_meas_true : Outport  Port=12
  wires:
  Three-axis Gyroscope/1 -> "Gyro, raw"/1
  Three-axis Accelerometer/1 -> "Accel, raw"/1
  Plant/11(PQR) -> PQR_true/1, Three-axis Gyroscope/1
  Plant/14(Static) -> Static (Pa)/1
  Plant/8(GPS Lat (rad)) -> "GPS Lat, rad"/1
  Plant/9(GPS Long (rad)) -> "GPS Long, rad"/1
  Plant/10(GPS H (m)) -> "GPS H, m"/1
  Plant/20(Ab meas) -> Three-axis Accelerometer/1, Ab_meas_true/1
  Plant/21(Vb) -> V_b_true/1
  Plant/15(Euler) -> Euler_true (rad)/1
  Plant/18(Vned) -> Vned_true/1
  Plant/1(GPS Month) -> Terminator11/1
  Plant/2(GPS Day) -> Terminator2/1
  Plant/3(GPS Year) -> Terminator3/1
  Plant/4(GPS Hr) -> Terminator1/1
  Plant/5(GPS Min) -> Terminator9/1
  Plant/6(GPS Sec) -> Terminator10/1
  Plant/7(GPS Frac Sec) -> Terminator12/1
  Plant/12(Ab) -> Terminator13/1
  Plant/13(Dynamic) -> Terminator14/1
  Plant/16(Vmag) -> Terminator15/1
  Plant/17(RPM) -> Terminator16/1
  Plant/19(aoa/betta,deg) -> Terminator17/1
  de,rad/1 -> Angle Conversion/1
  da,rad/1 -> Angle Conversion1/1
  "dr, rad"/1 -> Angle Conversion2/1
  dt/1 -> Plant/4(dt)
  "df, rad"/1 -> Angle Conversion3/1
  Angle Conversion/1 -> Plant/1(de)
  Angle Conversion1/1 -> Plant/2(da)
  Angle Conversion2/1 -> Plant/3(dr)
  Angle Conversion3/1 -> Plant/5(df)
  Plant/22(Euler_dot) -> Euler_dot_true/1

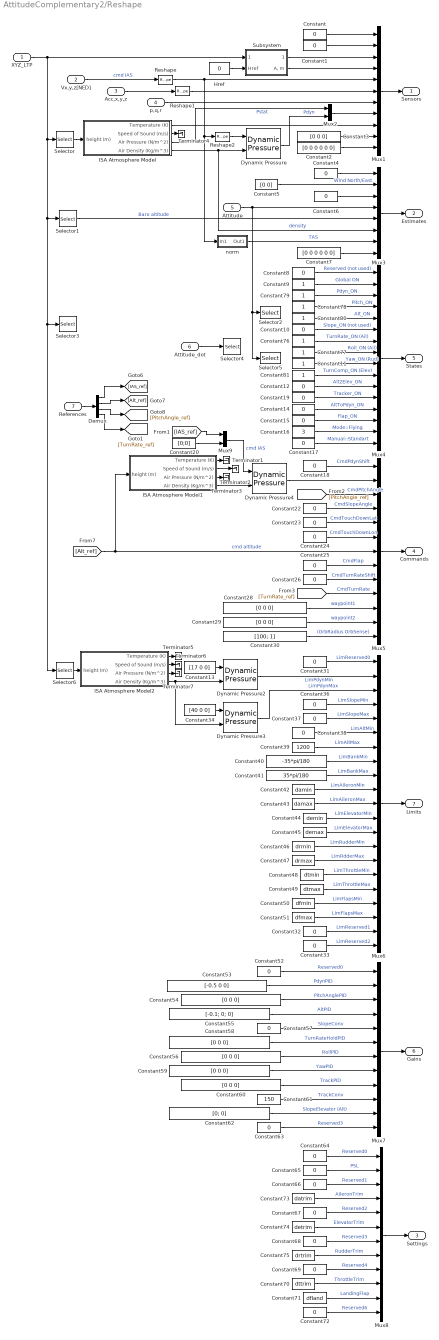
== system AttitudeComplementary2/Reshape ==
  XYZ_LTP : Inport  OutDataType=fixdt(1,16,0)  OutScaling=[]
  Vx,y,z[NED] : Inport  Port=2  OutDataType=fixdt(1,16,0)  OutScaling=[]
  Acc,x,y,z : Inport  Port=3  OutDataType=fixdt(1,16,0)  OutScaling=[]
  p,q,r : Inport  Port=4  OutDataType=fixdt(1,16,0)  OutScaling=[]
  Attitude : Inport  Port=5  OutDataType=fixdt(1,16,0)  OutScaling=[]
  Attitude_dot : Inport  Port=6  OutDataType=fixdt(1,16,0)  OutScaling=[]
  References : Inport  Port=7  OutDataType=fixdt(1,16,0)  OutScaling=[]
  Constant{,1,4,6,8,10,12,14..15,17..19,22..26,31..33,36..38,52,57,63..69,72} (33 alike) : Constant  Value=0
  Constant{9,11,76..81} (8 alike) : Constant
  Constant13 : Constant  Value=[17 0 0]
  Constant16 : Constant  Value=3
  Constant2 : Constant  Value=[0 0 0 0 0 0]
  Constant20 : Constant  Value=[0;0]
  Constant{3,28..29,54,56,58..60} (8 alike) : Constant  Value=[0 0 0]
  Constant30 : Constant  Value=[100; 1]
  Constant34 : Constant  Value=[40 0 0]
  Constant39 : Constant  Value=1200
  Constant40 : Constant  Value=-35*pi/180
  Constant41 : Constant  Value=35*pi/180
  Constant42 : Constant  Value=damin
  Constant43 : Constant  Value=damax
  Constant44 : Constant  Value=demin
  Constant45 : Constant  Value=demax
  Constant46 : Constant  Value=drmin
  Constant47 : Constant  Value=drmax
  Constant48 : Constant  Value=dtmin
  Constant49 : Constant  Value=dtmax
  Constant5 : Constant  Value=[0 0]
  Constant50 : Constant  Value=dfmin
  Constant51 : Constant  Value=dfmax
  Constant53 : Constant  Value=[-0.5 0 0]
  Constant55 : Constant  Value=[-0.1; 0; 0]
  Constant61 : Constant  Value=150
  Constant62 : Constant  Value=[0; 0]
  Constant7 : Constant  Value=[0 0 0 0 0 0]
  Constant70 : Constant  Value=dttrim
  Constant71 : Constant  Value=dfland
  Constant73 : Constant  Value=datrim
  Constant74 : Constant  Value=detrim
  Constant75 : Constant  Value=drtrim
  Demux : Demux
  Dynamic Pressure{,2..4} (4 alike) : aerolibasang/Dynamic Pressure  SystemSampleTime=-1
  Href : Constant  Value=0
  ISA Atmosphere Model : Subsystem  mask(International Standart Atmosphere){L=ISA_lapse, h_lim=ISA_hmax, R=ISA_R, g=ISA_g, rh0=ISA_rho0, P0=ISA_P0, T0=ISA_T0}
      mask prompts: L "Lapse rate"; h_lim "Upper altitude limit, (m)"; R "Universal gas constant R"; g "Garvity constant, (m/c^2)"; rh0 "Sea level density, (kg/m^3)"; P0 "Sea level pressure, (N/m^2)"; T0 "Sea level temperature, (K)"
  ISA Atmosphere Model1 : Subsystem  mask(International Standart Atmosphere){L=ISA_lapse, h_lim=ISA_hmax, R=ISA_R, g=ISA_g, rh0=ISA_rho0, P0=ISA_P0, T0=ISA_T0}
      mask prompts: L "Lapse rate"; h_lim "Upper altitude limit, (m)"; R "Universal gas constant R"; g "Garvity constant, (m/c^2)"; rh0 "Sea level density, (kg/m^3)"; P0 "Sea level pressure, (N/m^2)"; T0 "Sea level temperature, (K)"
  ISA Atmosphere Model2 : Subsystem  mask(International Standart Atmosphere){L=ISA_lapse, h_lim=ISA_hmax, R=ISA_R, g=ISA_g, rh0=ISA_rho0, P0=ISA_P0, T0=ISA_T0}
      mask prompts: L "Lapse rate"; h_lim "Upper altitude limit, (m)"; R "Universal gas constant R"; g "Garvity constant, (m/c^2)"; rh0 "Sea level density, (kg/m^3)"; P0 "Sea level pressure, (N/m^2)"; T0 "Sea level temperature, (K)"
  Mux1 : Mux  Inputs=11
  Mux2 : Mux  Inputs=2
  Mux3 : Mux  Inputs=8
  Mux4 : Mux  Inputs=16
  Mux5 : Mux  Inputs=13
  Mux6 : Mux  Inputs=21
  Mux7 : Mux  Inputs=12
  Mux8 : Mux  Inputs=12
  Mux9 : Mux  Inputs=2
  Reshape : Reshape
  Reshape1 : Reshape
  Reshape2 : Reshape
  Selector{,1,3..4,6} (5 alike) : Selector  IndexOptions=Index vector (dialog)  Indices=3  OutputSizes=[(-2)]  InputPortWidth=3
  Selector2 : Selector  IndexOptions=Index vector (dialog)  Indices=2  OutputSizes=[(-2)]  InputPortWidth=3
  Selector5 : Selector  IndexOptions=Index vector (dialog)  Indices=[1 3]  OutputSizes=[(-2)]  InputPortWidth=3
  Subsystem : Subsystem
  Terminator{1..7} (7 alike) : Terminator
  norm : Subsystem
  Sensors : Outport  OutDataType=fixdt(1,16,0)  OutScaling=[]
  Estimates : Outport  Port=2  OutDataType=fixdt(1,16,0)  OutScaling=[]
  Settings : Outport  Port=3  OutDataType=fixdt(1,16,0)  OutScaling=[]
  Commands : Outport  Port=4  OutDataType=fixdt(1,16,0)  OutScaling=[]
  States : Outport  Port=5  OutDataType=fixdt(1,16,0)  OutScaling=[]
  Gains : Outport  Port=6  OutDataType=fixdt(1,16,0)  OutScaling=[]
  Limits : Outport  Port=7  OutDataType=fixdt(1,16,0)  OutScaling=[]
  wires:
  Constant/1 -> Mux1/1
  Constant1/1 -> Mux1/2
  Subsystem/1("LL, deg") -> Mux1/3
  Subsystem/2("A, m") -> Mux1/4
  XYZ_LTP/1 -> Subsystem/1("XYZ, ltp"), Selector/1, Selector1/1, Selector3/1, Selector6/1
  Vx,y,z[NED]/1 -> Reshape/1  "cmd IAS"
  Mux1/1 -> Sensors/1
  Acc,x,y,z/1 -> Reshape1/1
  p,q,r/1 -> Mux1/7
  Constant3/1 -> Mux1/10
  Constant2/1 -> Mux1/11
  ISA Atmosphere Model/4(Air Density (Kg/m^3)) -> Dynamic Pressure/2, Mux3/6  "density"
  ISA Atmosphere Model/1(Temperature (K)) -> Mux1/9
  Mux2/1 -> Mux1/8
  ISA Atmosphere Model/3("Air Pressure (N/m^2) ") -> Mux2/1  "Pstat"
  ISA Atmosphere Model/2("Speed of Sound (m/s) ") -> Terminator4/1
  Dynamic Pressure/1 -> Mux2/2  "Pdyn"
  Selector/1 -> ISA Atmosphere Model/1(height (m))
  Reshape/1 -> Mux1/5, Reshape2/1, norm/1(In1)
  Reshape1/1 -> Mux1/6
  Reshape2/1 -> Dynamic Pressure/1
  Href/1 -> Subsystem/2(Href)
  Mux3/1 -> Estimates/1
  Constant4/1 -> Mux3/1
  Constant5/1 -> Mux3/2  "Wind North/East"
  Constant6/1 -> Mux3/3
  Attitude/1 -> Selector2/1, Selector5/1, Mux3/4
  Selector1/1 -> Mux3/5  "Baro altitude"
  norm/1(Out1) -> Mux3/7  "TAS"
  Constant7/1 -> Mux3/8
  Mux4/1 -> States/1
  Constant8/1 -> Mux4/1  "Reserved (not used)"
  Constant9/1 -> Mux4/2  "Global ON"
  Constant10/1 -> Mux4/6  "Slope_ON (not used)"
  Attitude_dot/1 -> Selector4/1
  Constant11/1 -> Mux4/9  "Yaw_ON (Rud)"
  Mux5/1 -> Commands/1
  Constant18/1 -> Mux5/1  "CmdPdynShift"
  ISA Atmosphere Model1/1(Temperature (K)) -> Terminator1/1
  ISA Atmosphere Model1/2("Speed of Sound (m/s) ") -> Terminator2/1
  ISA Atmosphere Model1/3("Air Pressure (N/m^2) ") -> Terminator3/1
  ISA Atmosphere Model1/4(Air Density (Kg/m^3)) -> Dynamic Pressure4/2
  Dynamic Pressure4/1 -> Mux5/2
  Mux9/1 -> Dynamic Pressure4/1  "cmd IAS"
  [Alt_ref] -> ISA Atmosphere Model1/1(height (m)), Mux5/7  "cmd altitude"
  [PitchAngle_ref] -> Mux5/3  "CmdPitchAngle"
  Constant22/1 -> Mux5/4  "CmdSlopeAngle"
  Constant24/1 -> Mux5/6  "CmdTouchDownLon"
  Constant23/1 -> Mux5/5  "CmdTouchDownLat"
  Constant25/1 -> Mux5/8  "CmdFlap"
  Constant26/1 -> Mux5/9  "CmdTurnRateShift"
  [TurnRate_ref] -> Mux5/10  "CmdTurnRate"
  Constant28/1 -> Mux5/11  "waypoint1"
  Constant29/1 -> Mux5/12  "waypoint2"
  Constant30/1 -> Mux5/13  "(OrbRadius OrbSense)"
  Mux6/1 -> Limits/1
  Constant31/1 -> Mux6/1  "LimReserved0"
  Constant33/1 -> Mux6/21  "LimReserved2"
  Constant32/1 -> Mux6/20  "LimReserved1"
  ISA Atmosphere Model2/1(Temperature (K)) -> Terminator5/1
  ISA Atmosphere Model2/2("Speed of Sound (m/s) ") -> Terminator6/1
  ISA Atmosphere Model2/3("Air Pressure (N/m^2) ") -> Terminator7/1
  ISA Atmosphere Model2/4(Air Density (Kg/m^3)) -> Dynamic Pressure2/2, Dynamic Pressure3/2
  Constant13/1 -> Dynamic Pressure2/1
  Constant34/1 -> Dynamic Pressure3/1
  Selector6/1 -> ISA Atmosphere Model2/1(height (m))
  Dynamic Pressure2/1 -> Mux6/2  "LimPdynMin"
  Dynamic Pressure3/1 -> Mux6/3  "LimPdynMax"
  Constant36/1 -> Mux6/4  "LimSlopeMin"
  Constant37/1 -> Mux6/5  "LimSlopeMax"
  Constant38/1 -> Mux6/6  "LimAltMin"
  Constant39/1 -> Mux6/7  "LimAltMax"
  Constant40/1 -> Mux6/8  "LimBankMin"
  Constant41/1 -> Mux6/9  "LimBankMax"
  Constant42/1 -> Mux6/10  "LimAileronMin"
  Constant43/1 -> Mux6/11  "LimAileronMax"
  Constant44/1 -> Mux6/12  "LimElevatorMin"
  Constant45/1 -> Mux6/13  "LimElevatorMax"
  Constant46/1 -> Mux6/14  "LimRudderMin"
  Constant47/1 -> Mux6/15  "LimRdderMax"
  Constant48/1 -> Mux6/16  "LimThrottleMin"
  Constant49/1 -> Mux6/17  "LimThrottleMax"
  Constant50/1 -> Mux6/18  "LimFlapsMin"
  Constant51/1 -> Mux6/19  "LimFlapsMax"
  Mux7/1 -> Gains/1
  Constant52/1 -> Mux7/1  "Reserved0"
  Constant53/1 -> Mux7/2  "PdynPID"
  Constant54/1 -> Mux7/3  "PitchAnglePID"
  Constant55/1 -> Mux7/4  "AltPID"
  Constant58/1 -> Mux7/6  "TurnRateHoldPID"
  Constant57/1 -> Mux7/5  "SlopeConv"
  Constant56/1 -> Mux7/7  "RollPID"
  Constant59/1 -> Mux7/8  "YawPID"
  Constant60/1 -> Mux7/9  "TrackPID"
  Constant61/1 -> Mux7/10  "TrackConv"
  Constant62/1 -> Mux7/11  "SlopeElevator (Alt)"
  Constant63/1 -> Mux7/12  "Reserved3"
  Mux8/1 -> Settings/1
  Constant64/1 -> Mux8/1  "Reserved0"
  Constant65/1 -> Mux8/2  "PSL"
  Constant66/1 -> Mux8/3  "Reserved1"
  Constant67/1 -> Mux8/5  "Reserved2"
  Constant68/1 -> Mux8/7  "Reserved3"
  Constant69/1 -> Mux8/9  "Reserved4"
  Constant70/1 -> Mux8/10  "ThrottleTrim"
  Constant71/1 -> Mux8/11  "LandingFlap"
  Constant72/1 -> Mux8/12  "Reserved6"
  Constant73/1 -> Mux8/4  "AileronTrim"
  Constant74/1 -> Mux8/6  "ElevatorTrim"
  Constant75/1 -> Mux8/8  "RudderTrim"
  Constant76/1 -> Mux4/7  "TurnRate_ON (Ail)"
  Constant77/1 -> Mux4/8  "Roll_ON (Ail)"
  Constant78/1 -> Mux4/4  "Pitch_ON"
  Constant79/1 -> Mux4/3  "Pdyn_ON"
  Constant80/1 -> Mux4/5  "Alt_ON"
  Constant81/1 -> Mux4/10  "TurnComp_ON (Elev)"
  Constant12/1 -> Mux4/11  "Alt2Elev_ON"
  Constant19/1 -> Mux4/12  "Tracker_ON"
  Constant14/1 -> Mux4/13  "AltToPdyn_ON"
  Constant15/1 -> Mux4/14  "Flap_ON"
  Constant16/1 -> Mux4/15  "Mode::Flying"
  Constant17/1 -> Mux4/16  "Manual::Standart"
  References/1 -> Demux/1
  Demux/1 -> [IAS_ref]
  Demux/2 -> [Alt_ref]
  Demux/3 -> [PitchAngle_ref]
  Demux/4 -> [TurnRate_ref]
  Constant20/1 -> Mux9/2
  [IAS_ref] -> Mux9/1

== system AttitudeComplementary2/Signal Cond ==
  G_raw : Inport
  A_raw : Inport  Port=2
  Accel Convert : Subsystem
  Gyro Convert : Subsystem
  PQR_sen : Outport
  A_sens : Outport  Port=2
  wires:
  G_raw/1 -> Gyro Convert/1(Raw)
  Gyro Convert/1(Comp) -> PQR_sen/1
  A_raw/1 -> Accel Convert/1(Raw)
  Accel Convert/1(Comp) -> A_sens/1

== system AttitudeComplementary2/Subsystem ==
  PQR_t : Inport
  PQR_h : Inport  Port=2
  Angle Conversion1 : aerolibconvert2/Angle Conversion  SystemSampleTime=-1  IU=rad  OU=deg
  Angle Conversion5 : aerolibconvert2/Angle Conversion  SystemSampleTime=-1  IU=rad  OU=deg
  Angle Conversion6 : aerolibconvert2/Angle Conversion  SystemSampleTime=-1  IU=rad  OU=deg
  Sum2 : Sum  Inputs=+-|
  PQR_t,deg : Outport
  PQR_h,deg : Outport  Port=2
  PQR_err,deg : Outport  Port=3
  wires:
  PQR_t/1 -> Angle Conversion6/1, Sum2/1
  PQR_h/1 -> Angle Conversion1/1, Sum2/2
  Sum2/1 -> Angle Conversion5/1
  Angle Conversion6/1 -> PQR_t,deg/1
  Angle Conversion1/1 -> PQR_h,deg/1
  Angle Conversion5/1 -> PQR_err,deg/1

== system AttitudeComplementary2/Subsystem1 ==
  Eul_t : Inport
  Eul_hat : Inport  Port=2
  Angle Conversion2 : aerolibconvert2/Angle Conversion  SystemSampleTime=-1  IU=rad  OU=deg
  Angle Conversion3 : aerolibconvert2/Angle Conversion  SystemSampleTime=-1  IU=rad  OU=deg
  Angle Conversion4 : aerolibconvert2/Angle Conversion  SystemSampleTime=-1  IU=rad  OU=deg
  Sum : Sum  Inputs=+-|
  "Eul_t, deg" : Outport
  "Eul_h, deg" : Outport  Port=2
  "Eul_err, deg" : Outport  Port=3
  wires:
  Eul_t/1 -> Sum/1, Angle Conversion4/1
  Eul_hat/1 -> Sum/2, Angle Conversion2/1
  Sum/1 -> Angle Conversion3/1
  Angle Conversion4/1 -> "Eul_t, deg"/1
  Angle Conversion2/1 -> "Eul_h, deg"/1
  Angle Conversion3/1 -> "Eul_err, deg"/1

== system AttitudeComplementary2/Subsystem2 ==
  XYZ_t : Inport
  XYZ_h : Inport  Port=2
  Sum1 : Sum  Inputs=+-|
  XYZ_t,ned : Outport
  "XYZ_h, ned" : Outport  Port=2
  XYZ_err : Outport  Port=3
  wires:
  XYZ_h/1 -> Sum1/2, "XYZ_h, ned"/1
  XYZ_t/1 -> Sum1/1, XYZ_t,ned/1
  Sum1/1 -> XYZ_err/1

== system AttitudeComplementary2/get Psi ==
  GPS Bus : Inport
  Bus Selector : BusSelector  OutputSignals=ydot,xdot
  Fcn1 : Fcn  Expr=atan2(u(1),u(2))
  Mux : Mux  Inputs=2
  Psi : Outport
  wires:
  Fcn1/1 -> Psi/1
  GPS Bus/1 -> Bus Selector/1
  Bus Selector/2 -> Mux/2  "<xdot>"
  Bus Selector/1 -> Mux/1  "<ydot>"
  Mux/1 -> Fcn1/1

== system AttitudeComplementary2/Accel Comp/Get Roll, Pitch2 ==
  Ab : Inport
  Fcn : Fcn  Expr=atan(u(1)/-u(3))
  Fcn1 : Fcn  Expr=atan(u(2)/-u(3))
  Mux : Mux  Inputs=2
  "Phi, The" : Outport
  wires:
  Fcn1/1 -> Mux/1
  Fcn/1 -> Mux/2
  Ab/1 -> Fcn1/1, Fcn/1
  Mux/1 -> "Phi, The"/1

== system AttitudeComplementary2/Accel Comp/Gravity in {B} ==
  RLTP2B : Inport  Orientation=left
  "Gravity {I}" : Constant  Orientation=left  Value=[0 0 ISA_g]
  Product1 : Product  Orientation=left  Multiplication=Matrix(*)  RndMeth=Zero
  g_b : Outport  Orientation=left
  wires:
  "Gravity {I}"/1 -> Product1/2
  RLTP2B/1 -> Product1/1
  Product1/1 -> g_b/1

== system AttitudeComplementary2/Accel Comp/Subsystem ==
  Euler_hat : Inport  Orientation=left
  Vned : Inport  Orientation=left  Port=2
  Clock : Clock
  Constant : Constant  Orientation=left  Value=[0;0;0]
  Integer Delay2 : simulink/Discrete/Integer Delay  Orientation=left  vinit=0.0  samptime=-1  NumDelays=1
  LTP2B : dspmtrx3/Transpose  Orientation=left  SystemSampleTime=-1  Hermitian=off  overflowFlag=off
  Product : Product  Orientation=left  Multiplication=Matrix(*)  RndMeth=Zero
  RB2LTP : Subsystem  Orientation=left
  Switch : Switch  Orientation=left  Criteria=u2 > Threshold
  Vb_gps : Outport  Orientation=left
  RB2LT : Outport  Orientation=left  Port=2
  RLT2B : Outport  Orientation=left  Port=3
  wires:
  Euler_hat/1 -> Integer Delay2/1
  Integer Delay2/1 -> RB2LTP/1(Euler)
  LTP2B/1 -> Product/1, RLT2B/1
  Vned/1 -> Product/2
  RB2LTP/1(Rot) -> LTP2B/1, RB2LT/1
  Switch/1 -> Vb_gps/1
  Product/1 -> Switch/1
  Clock/1 -> Switch/2
  Constant/1 -> Switch/3
